simulink model "SoC_Estimation_UKF_2RC"  (R2022b)
settings: Solver=FixedStepAuto  StartTime=0.0  StopTime=time(end)  FixedStep=0.1  MaxStep=1e-2  MinStep=1e-3  RelTol=1e-3
InitFcn:
  | %% Load Dataset
  | if(exist("Battery","var")==0 && exist("SOC_LUT","var")==0)
  | clc; clear variables;
  | [file,folder]=uigetfile('*.*','Select Data File');
  | path=fullfile(folder,file);
  | load(path);
  | if(exist("Robot","var")==1)
  |     Battery=Robot;
  | elseif(exist("meas","var")==1)
  |     Battery=meas;
  |     Battery.Capacity = 2.9;
  | end
  | 
  | 
  | [time, Ia, Ic] = unique(Battery.Time); % Delete duplicate time
  | voltage = Battery.Voltage(Ia);
  | current = Battery.Current(Ia);
  | Ah = Battery.Ah(Ia);
  | if(Ah(end)<0)
  |     Ah=-Ah;
  | end
  | if(mean(current)<0)
  | current = -current; % Discharge current must be positive
  | end
  | SOC_REAL = 1-Ah/Battery.Capacity; % Discharge current must be positive
  | 
  | initialPoint=1;
  | %% Load Parameters
  | [file,folder]=uigetfile('*.*','Select Parameter File');
  | path=fullfile(folder,file);
  | load(path);
  | end
model workspace (MAT data in the model file):
  R = 1.00050162835
values from neighbouring files (symbols this model uses):
  C1 = [118829.925056 7679.67487496 914.032998183 995.696239615 1030.86324658 8477.81093389 1000000 8701.64070127 913.695760467 229.654526583]    [LFP_2RC_Parameters_PSO_13_10_2023_17_30.mat]    (also in LFP_2RC_Parameters_PSO_18_10_2023_15_27.mat = [374.526915394 91616.0371283 413980.590037 980.096839909 464; LFP_2RC_Parameters_PSO_18_10_2023_15_38.mat = [146.566073865 937.05567026 992.511993063 1291.92677117 1452; LFP_2RC_Parameters_PSO_18_10_2023_15_46.mat = [4572764.90937 926.813715587 992.544001108 773.772276009 111; NMC_2RC_Parameters_PSO_11_09_2023_10_18.mat = [27.3638316243 1000 21.9335529229 1000 31.8018075879 26.2311)
  C2 = [7193.14418842 3500000 13830.314823 10815.547426 12725.8630835 2986560.60044 129.09603881 93182.2545509 10234.9855741 3500000]    [LFP_2RC_Parameters_PSO_13_10_2023_17_30.mat]    (also in LFP_2RC_Parameters_PSO_18_10_2023_15_27.mat = [8152.77757794 7772.75056844 32340.9237315 10784.3399167 103; LFP_2RC_Parameters_PSO_18_10_2023_15_38.mat = [5380.51009562 16240.5476942 16189.4861318 10368.8792756 134; LFP_2RC_Parameters_PSO_18_10_2023_15_46.mat = [5339.98210013 16310.3382976 16188.61063 8488.61060912 12765; NMC_2RC_Parameters_PSO_11_09_2023_10_18.mat = [1323.01639542 100 1413.11035886 100 1348.21886578 1246.8775)
  OCV = [12.860136 13.025615 13.131995 13.155635 13.161545 13.173365 13.232465 13.309296 13.309296 13.604795]    [LFP_2RC_Parameters_PSO_13_10_2023_17_30.mat]    (also in LFP_2RC_Parameters_PSO_18_10_2023_15_27.mat; LFP_2RC_Parameters_PSO_18_10_2023_15_38.mat; LFP_2RC_Parameters_PSO_18_10_2023_15_46.mat; NMC_2RC_Parameters_PSO_11_09_2023_10_18.mat = [3.21503 3.23112 3.23691 3.33792 3.34178 3.34436 3.345 3.366)
  R1 = [0.001 0.113528547574 0.0897221455408 0.0815153824808 0.073763090009 0.0722149483866 0.001 0.114920856231 0.0843574753205 0.170448149157]    [LFP_2RC_Parameters_PSO_13_10_2023_17_30.mat]    (also in LFP_2RC_Parameters_PSO_18_10_2023_15_27.mat = [0.130840731393 0.001 0.001 0.0812887278858 0.0893662319552 ; LFP_2RC_Parameters_PSO_18_10_2023_15_38.mat = [0.125407853943 0.106716849555 0.100754450021 0.077403767946; LFP_2RC_Parameters_PSO_18_10_2023_15_46.mat = [1e-05 0.107896547406 0.100751200842 0.0796558546904 0.06941; NMC_2RC_Parameters_PSO_11_09_2023_10_18.mat = [0.0786652045966 0.0830695574623 0.102018078057 0.0293575040)
  R2 = [0.327796783258 0.001 0.0807740022148 0.121640548886 0.0769058248858 0.001 0.248251890874 0.001 0.101537896805 0.001]    [LFP_2RC_Parameters_PSO_13_10_2023_17_30.mat]    (also in LFP_2RC_Parameters_PSO_18_10_2023_15_27.mat = [0.32439345834 0.113786678529 0.108222017066 0.121707134426 ; LFP_2RC_Parameters_PSO_18_10_2023_15_38.mat = [0.650495945143 0.197605258421 0.107392740699 0.095938803423; LFP_2RC_Parameters_PSO_18_10_2023_15_46.mat = [0.655432908645 0.19766392139 0.107391796285 0.103804820932 ; NMC_2RC_Parameters_PSO_11_09_2023_10_18.mat = [0.155221398827 0.0699206176425 0.18163313418 0.019432263083)
  Rt = [0.226652153247 0.225527584096 0.15909738837 0.148852656484 0.143946466873 0.188428407135 0.001 0.211746487785 0.13044097603 0.184475294934]    [LFP_2RC_Parameters_PSO_13_10_2023_17_30.mat]    (also in LFP_2RC_Parameters_PSO_18_10_2023_15_27.mat = [0.109760248591 0.225130502849 0.260964397417 0.148857487521; LFP_2RC_Parameters_PSO_18_10_2023_15_38.mat = [0.0991776836505 0.174037973313 0.155548900057 0.15434594036; LFP_2RC_Parameters_PSO_18_10_2023_15_46.mat = [0.222188102228 0.173070428684 0.155550513123 0.142559241614; NMC_2RC_Parameters_PSO_11_09_2023_10_18.mat = [0.0538374601523 0.0958739914905 0.0468761371301 0.053958081)
  SOC_INTP = 0:1/66:1    [Pestimation_PSO.m]
  SOC_LUT = [0.242928992505 0.325332427039 0.408229233889 0.491515232404 0.575389970179 0.659581229809 0.744212711848 0.829280881109 0.914612975737 1]    [LFP_2RC_Parameters_PSO_13_10_2023_17_30.mat]    (also in LFP_2RC_Parameters_PSO_18_10_2023_15_27.mat; LFP_2RC_Parameters_PSO_18_10_2023_15_38.mat; LFP_2RC_Parameters_PSO_18_10_2023_15_46.mat; NMC_2RC_Parameters_PSO_11_09_2023_10_18.mat = [0.0458068965517 0.0486103448276 0.0499965517241 0.090272413)
libraries: sharedTrackingLibrary x1
settings Model: Creator=monsalve  LastModifiedBy=monsalve
settings DataIOCC: ExternalInput=[time, current],[time,voltage], [time, Ah]  LoadExternalInput=on
settings DebuggingCC: UnconnectedInputMsg=warning  UnconnectedOutputMsg=warning  UnconnectedLineMsg=warning
settings ModelReferenceCC: EnableRefExpFcnMdlSchedulingChecks=on
settings RTWCC: DLArmComputeVersion=19.05

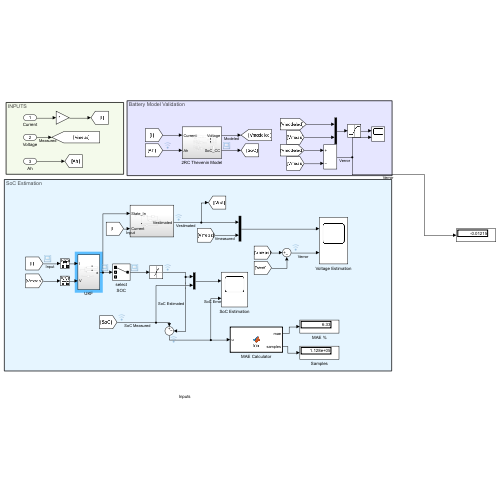
[thumbnail: Simulink's stored preview of the top-level diagram]
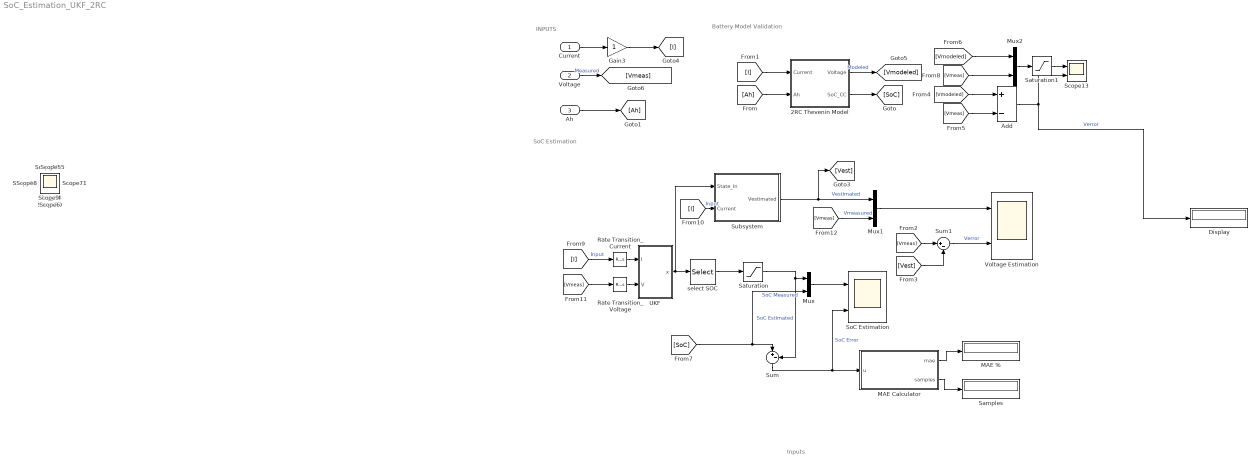
== system SoC_Estimation_UKF_2RC ==
  note: Inputs
  note: INPUTS
  note: Battery Model Validation
  note: SoC Estimation
  Current : Inport
  Voltage : Inport  Port=2
  Ah : Inport  Port=3
  2RC Thevenin Model : Subsystem
  Add : Sum  Inputs=+-
  Display : Display
  Gain3 : Gain
  MAE % : Display
  MAE Calculator : MATLAB Function  TreatAsAtomicUnit=on
  Mux : Mux  Inputs=2
  Mux1 : Mux  Inputs=2
  Mux2 : Mux  Inputs=2
  Rate Transition_Current : RateTransition  OutPortSampleTime=0.1
  Rate Transition_Voltage : RateTransition  InitialCondition=12  OutPortSampleTime=0.1
  Samples : Display
  Saturation : Saturate  UpperLimit=1  LowerLimit=0
  Saturation1 : Saturate  UpperLimit=5
  Scope13 : Scope  NumInputPorts=2
  SoC Estimation : Scope  NumInputPorts=2
  Subsystem : Subsystem
  Sum : Sum  Inputs=|+-
  Sum1 : Sum  Inputs=|+-
  UKF : Subsystem
  Voltage Estimation : Scope  NumInputPorts=2
  select SOC : Selector  InputPortWidth=3  IndexOptions=Index vector (dialog)  Indices=1  OutputSizes=1
  Scope{,1..12,14..21} (21 alike) : Scope
  wires:
  Rate Transition_Voltage/1 -> UKF/2(V)
  UKF/1(x) -> select SOC/1, Subsystem/1(State_In)
  select SOC/1 -> Saturation/1
  Sum/1 -> SoC Estimation/2, MAE Calculator/1(u)  "SoC Error"
  Mux1/1 -> Voltage Estimation/1
  Mux/1 -> SoC Estimation/1
  Saturation/1 -> Mux/1, Sum/2  "SoC Estimated"
  [I] -> Subsystem/2(Current)  "Input"
  MAE Calculator/1(mae) -> MAE %/1
  MAE Calculator/2(samples) -> Samples/1
  Subsystem/1(Vestimated) -> Mux1/1, [Vest]  "Vestimated"
  [Vmeas] -> Mux1/2  "Vmeasured"
  [Vmeas] -> Sum1/1
  [Vest] -> Sum1/2
  Sum1/1 -> Voltage Estimation/2  "Verror"
  [SoC] -> Sum/1, Mux/2  "SoC Measured"
  Rate Transition_Current/1 -> UKF/1(I)
  [Vmeas] -> Rate Transition_Voltage/1
  2RC Thevenin Model/1(Voltage) -> [Vmodeled]  "Modeled"
  [I] -> 2RC Thevenin Model/1(Current)
  Current/1 -> Gain3/1
  Gain3/1 -> [I]
  [Vmodeled] -> Add/1
  Mux2/1 -> Saturation1/1
  Voltage/1 -> [Vmeas]  "Measured"
  [Vmeas] -> Add/2
  [Vmodeled] -> Mux2/1
  2RC Thevenin Model/2(SoC_CC) -> [SoC]
  [Vmeas] -> Mux2/2
  Ah/1 -> [Ah]
  [Ah] -> 2RC Thevenin Model/2(Ah)
  [I] -> Rate Transition_Current/1  "Input"
  Add/1 -> Scope13/2, Display/1  "Verror"
  Saturation1/1 -> Scope13/1

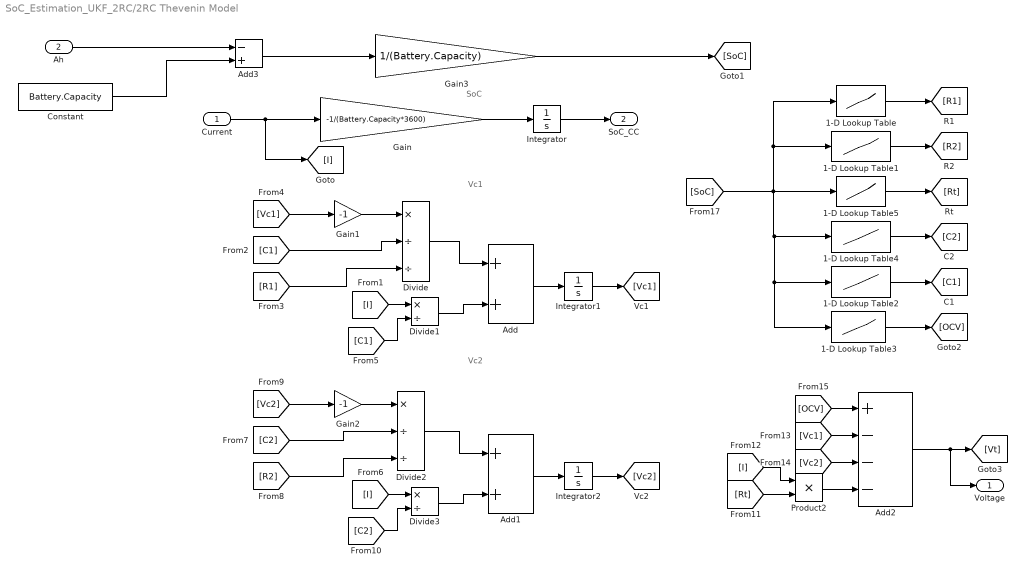
== system SoC_Estimation_UKF_2RC/2RC Thevenin Model ==
  note: Vc1
  note: SoC
  note: Vc2
  Current : Inport
  Ah : Inport  Port=2
  1-D Lookup Table : Lookup_n-D  NumberOfTableDimensions=1  BreakpointsForDimension1=SOC_LUT  Table=R1  InternalRulePriority=Speed  RndMeth=Simplest
  1-D Lookup Table1 : Lookup_n-D  NumberOfTableDimensions=1  BreakpointsForDimension1=SOC_LUT  Table=R2  InternalRulePriority=Speed  RndMeth=Simplest
  1-D Lookup Table2 : Lookup_n-D  NumberOfTableDimensions=1  BreakpointsForDimension1=SOC_LUT  Table=C1  InternalRulePriority=Speed  RndMeth=Simplest
  1-D Lookup Table3 : Lookup_n-D  NumberOfTableDimensions=1  BreakpointsForDimension1=SOC_INTP  Table=OCV  InternalRulePriority=Speed  RndMeth=Simplest
  1-D Lookup Table4 : Lookup_n-D  NumberOfTableDimensions=1  BreakpointsForDimension1=SOC_LUT  Table=C2  InternalRulePriority=Speed  RndMeth=Simplest
  1-D Lookup Table5 : Lookup_n-D  NumberOfTableDimensions=1  BreakpointsForDimension1=SOC_LUT  Table=Rt  InternalRulePriority=Speed  RndMeth=Simplest
  Add : Sum
  Add1 : Sum
  Add2 : Sum  Inputs=+---
  Add3 : Sum  Inputs=-+
  Constant : Constant  Value=Battery.Capacity
  Divide : Product  Inputs=*//
  Divide1 : Product  Inputs=*/
  Divide2 : Product  Inputs=*//
  Divide3 : Product  Inputs=*/
  Gain : Gain  Gain=-1/(Battery.Capacity*3600)
  Gain1 : Gain  Gain=-1
  Gain2 : Gain  Gain=-1
  Gain3 : Gain  Gain=1/(Battery.Capacity)
  Integrator : Integrator  InitialCondition=1  LimitOutput=on  UpperSaturationLimit=1  LowerSaturationLimit=0
  Integrator1 : Integrator
  Integrator2 : Integrator
  Product2 : Product
  Voltage : Outport
  SoC_CC : Outport  Port=2
  wires:
  Product2/1 -> Add2/4
  Add1/1 -> Integrator2/1
  1-D Lookup Table4/1 -> [C2]
  [SoC] -> 1-D Lookup Table3/1, 1-D Lookup Table2/1, 1-D Lookup Table4/1, 1-D Lookup Table5/1, 1-D Lookup Table1/1, 1-D Lookup Table/1
  [OCV] -> Add2/1
  [R1] -> Divide/3
  Divide1/1 -> Add/2
  Integrator2/1 -> [Vc2]
  [Vc1] -> Gain1/1
  Divide3/1 -> Add1/2
  Add/1 -> Integrator1/1
  Divide/1 -> Add/1
  1-D Lookup Table/1 -> [R1]
  Gain/1 -> Integrator/1
  [I] -> Divide3/1
  1-D Lookup Table3/1 -> [OCV]
  1-D Lookup Table2/1 -> [C1]
  [Vc2] -> Add2/3
  [C2] -> Divide2/2
  [Rt] -> Product2/2
  Add2/1 -> Voltage/1, [Vt]
  [I] -> Divide1/1
  [I] -> Product2/1
  Divide2/1 -> Add1/1
  [R2] -> Divide2/3
  1-D Lookup Table5/1 -> [Rt]
  Current/1 -> [I], Gain/1
  [C1] -> Divide/2
  [C2] -> Divide3/2
  1-D Lookup Table1/1 -> [R2]
  Gain2/1 -> Divide2/1
  [Vc2] -> Gain2/1
  Gain1/1 -> Divide/1
  [Vc1] -> Add2/2
  Integrator1/1 -> [Vc1]
  Integrator/1 -> SoC_CC/1
  [C1] -> Divide1/2
  Ah/1 -> Add3/1
  Add3/1 -> Gain3/1
  Constant/1 -> Add3/2
  Gain3/1 -> [SoC]

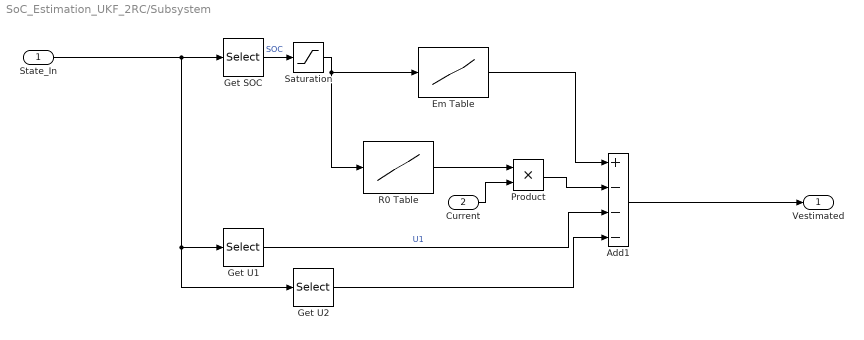
== system SoC_Estimation_UKF_2RC/Subsystem ==
  State_In : Inport
  Current : Inport  Port=2
  Add1 : Sum  Inputs=+---
  Em Table : Lookup_n-D  NumberOfTableDimensions=1  BreakpointsForDimension1=SOC_LUT  BreakpointsForDimension2=Battery.Temperature_LUT  Table=OCV  InternalRulePriority=Speed  RndMeth=Simplest
  Get SOC : Selector  InputPortWidth=3  IndexOptions=Index vector (dialog)  Indices=[1]  OutputSizes=1
  Get U1 : Selector  InputPortWidth=3  IndexOptions=Index vector (dialog)  Indices=2  OutputSizes=1
  Get U2 : Selector  InputPortWidth=3  IndexOptions=Index vector (dialog)  Indices=3  OutputSizes=1
  Product : Product
  R0 Table : Lookup_n-D  NumberOfTableDimensions=1  BreakpointsForDimension1=SOC_LUT  BreakpointsForDimension2=Battery.Temperature_LUT  Table=Rt  InternalRulePriority=Speed  RndMeth=Simplest
  Saturation : Saturate  UpperLimit=1  LowerLimit=0
  Vestimated : Outport
  wires:
  Current/1 -> Product/2
  R0 Table/1 -> Product/1
  Get U2/1 -> Add1/4
  Product/1 -> Add1/2
  Get U1/1 -> Add1/3  "U1"
  Em Table/1 -> Add1/1
  State_In/1 -> Get U2/1, Get U1/1, Get SOC/1
  Get SOC/1 -> Saturation/1  "SOC"
  Add1/1 -> Vestimated/1
  Saturation/1 -> R0 Table/1, Em Table/1

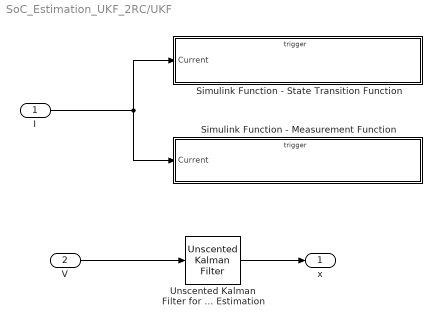
== system SoC_Estimation_UKF_2RC/UKF ==
  I : Inport
  V : Inport  Port=2
  Simulink Function - Measurement Function : Subsystem  TreatAsAtomicUnit=on
  Simulink Function - State Transition Function : Subsystem  TreatAsAtomicUnit=on
  Unscented Kalman Filter for SOC Estimation : sharedTrackingLibrary/Unscented Kalman Filter  StateTransitionFcn=batteryStateFcn  HasAdditiveProcessNoise=Additive  ProcessNoise=diag([1e-8,1e-8,1e-8])  HasTimeVaryingProcessNoise=off  HasStateTransitionFcnExtraArgument=0  InitialState=[1, 0, 0]  InitialStateCovariance=diag([1e-5,1,1])  Alpha=1  Beta=2  Kappa=0  MeasurementFcn1=batteryMeasurementFcn  HasMeasurementEnablePort1=off  HasAdditiveMeasurementNoise1=Additive  MeasurementNoise1=1  HasTimeVaryingMeasurementNoise1=off  HasMeasurementFcnExtraArgument1=0  HasMeasurementWrapping1=off  MeasurementFcn2=myMeasurementFcn  HasMeasurementEnablePort2=off  HasAdditiveMeasurementNoise2=Additive  MeasurementNoise2=1  HasTimeVaryingMeasurementNoise2=off  HasMeasurementFcnExtraArgument2=0  HasMeasurementWrapping2=off  MeasurementFcn3=myMeasurementFcn  HasMeasurementEnablePort3=off  HasAdditiveMeasurementNoise3=Additive  MeasurementNoise3=1  HasTimeVaryingMeasurementNoise3=off  HasMeasurementFcnExtraArgument3=0  HasMeasurementWrapping3=off  MeasurementFcn4=myMeasurementFcn  HasMeasurementEnablePort4=off  HasAdditiveMeasurementNoise4=Additive  MeasurementNoise4=1  HasTimeVaryingMeasurementNoise4=off  HasMeasurementFcnExtraArgument4=0  HasMeasurementWrapping4=off  MeasurementFcn5=myMeasurementFcn  HasMeasurementEnablePort5=off  HasAdditiveMeasurementNoise5=Additive  MeasurementNoise5=1  HasTimeVaryingMeasurementNoise5=off  HasMeasurementFcnExtraArgument5=0  HasMeasurementWrapping5=off  EnableMultirate=off  StateTransitionFcnSampleTime=-1  MeasurementFcn1SampleTime=-1  MeasurementFcn2SampleTime=-1  MeasurementFcn3SampleTime=-1  MeasurementFcn4SampleTime=-1  MeasurementFcn5SampleTime=-1  UseCurrentEstimator=on  OutputStateCovariance=off  DataType=double  SampleTime=0.1  NumberOfMeasurements=1
  x : Outport  VectorParamsAs1DForOutWhenUnconnected=off
  wires:
  I/1 -> Simulink Function - Measurement Function/1(Current), Simulink Function - State Transition Function/1(Current)
  V/1 -> Unscented Kalman Filter for SOC Estimation/1
  Unscented Kalman Filter for SOC Estimation/1 -> x/1

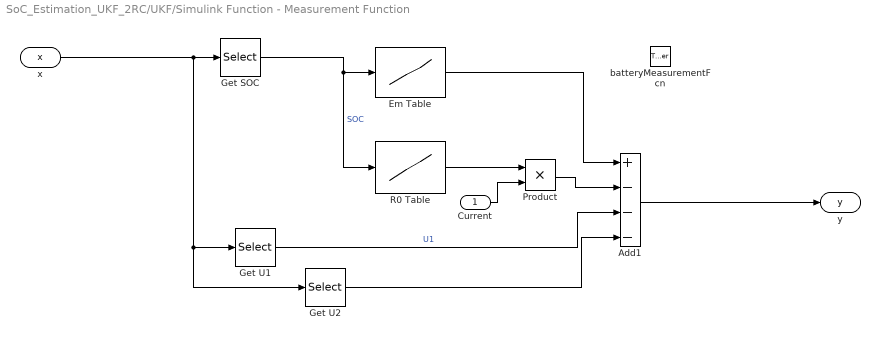
== system SoC_Estimation_UKF_2RC/UKF/Simulink Function - Measurement Function ==
  Current : Inport
  batteryMeasurementFcn : TriggerPort  TriggerType=function-call  IsSimulinkFunction=on  FunctionName=batteryMeasurementFcn  VariantControl=Variant
  Add1 : Sum  Inputs=+---
  Em Table : Lookup_n-D  NumberOfTableDimensions=1  BreakpointsForDimension1=SOC_LUT  BreakpointsForDimension2=Battery.Temperature_LUT  Table=OCV  InternalRulePriority=Speed  RndMeth=Simplest
  Get SOC : Selector  InputPortWidth=3  IndexOptions=Index vector (dialog)  Indices=[1]  OutputSizes=1
  Get U1 : Selector  InputPortWidth=3  IndexOptions=Index vector (dialog)  Indices=2  OutputSizes=1
  Get U2 : Selector  InputPortWidth=3  IndexOptions=Index vector (dialog)  Indices=3  OutputSizes=1
  Product : Product
  R0 Table : Lookup_n-D  NumberOfTableDimensions=1  BreakpointsForDimension1=SOC_LUT  BreakpointsForDimension2=Battery.Temperature_LUT  Table=Rt  InternalRulePriority=Speed  RndMeth=Simplest
  x : ArgIn  DisableCoverage=on  PortDimensions=3  ArgumentName=x
  y : ArgOut  DisableCoverage=on  ArgumentName=y
  wires:
  x/1 -> Get U2/1, Get U1/1, Get SOC/1
  Get SOC/1 -> R0 Table/1, Em Table/1  "SOC"
  Em Table/1 -> Add1/1
  R0 Table/1 -> Product/1
  Current/1 -> Product/2
  Product/1 -> Add1/2
  Get U1/1 -> Add1/3  "U1"
  Get U2/1 -> Add1/4
  Add1/1 -> y/1

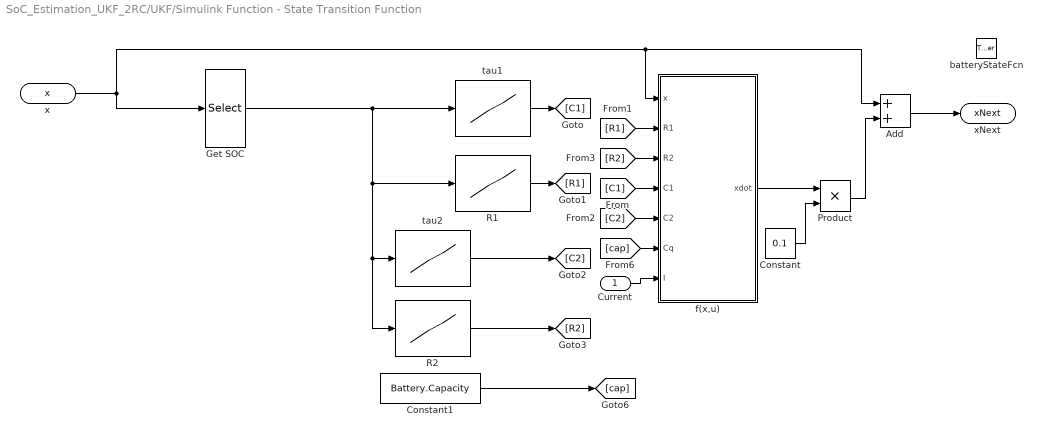
== system SoC_Estimation_UKF_2RC/UKF/Simulink Function - State Transition Function ==
  Current : Inport
  batteryStateFcn : TriggerPort  TriggerType=function-call  IsSimulinkFunction=on  FunctionName=batteryStateFcn  VariantControl=Variant
  Add : Sum
  Constant : Constant  Value=0.1
  Constant1 : Constant  Value=Battery.Capacity
  Get SOC : Selector  InputPortWidth=3  IndexOptions=Index vector (dialog)  Indices=1  OutputSizes=1
  Product : Product
  R1 : Lookup_n-D  NumberOfTableDimensions=1  BreakpointsForDimension1=SOC_LUT  BreakpointsForDimension2=Battery.Temperature_LUT  Table=R1  InternalRulePriority=Speed  RndMeth=Simplest
  R2 : Lookup_n-D  NumberOfTableDimensions=1  BreakpointsForDimension1=SOC_LUT  BreakpointsForDimension2=Battery.Temperature_LUT  Table=R2  InternalRulePriority=Speed  RndMeth=Simplest
  f(x,u) : MATLAB Function  TreatAsAtomicUnit=on
  tau1 : Lookup_n-D  NumberOfTableDimensions=1  BreakpointsForDimension1=SOC_LUT  BreakpointsForDimension2=Battery.Temperature_LUT  Table=C1  InternalRulePriority=Speed  RndMeth=Simplest
  tau2 : Lookup_n-D  NumberOfTableDimensions=1  BreakpointsForDimension1=SOC_LUT  BreakpointsForDimension2=Battery.Temperature_LUT  Table=C2  InternalRulePriority=Speed  RndMeth=Simplest
  x : ArgIn  DisableCoverage=on  PortDimensions=3  ArgumentName=x
  xNext : ArgOut  DisableCoverage=on  PortDimensions=3  ArgumentName=xNext
  wires:
  x/1 -> Get SOC/1, f(x,u)/1(x), Add/1
  Add/1 -> xNext/1
  Constant/1 -> Product/2
  f(x,u)/1(xdot) -> Product/1
  Product/1 -> Add/2
  tau1/1 -> [C1]
  [C1] -> f(x,u)/4(C1)
  R1/1 -> [R1]
  [R1] -> f(x,u)/2(R1)
  tau2/1 -> [C2]
  [C2] -> f(x,u)/5(C2)
  R2/1 -> [R2]
  [R2] -> f(x,u)/3(R2)
  Current/1 -> f(x,u)/7(I)
  Constant1/1 -> [cap]
  [cap] -> f(x,u)/6(Cq)
  Get SOC/1 -> R1/1, R2/1, tau2/1, tau1/1

== matlab function SoC_Estimation_UKF_2RC/MAE Calculator ==
  settings: updateMethod=DISCRETE
  data: u input; mae output; samples output
function [mae,samples]= fcn(u)
persistent sum i
if(isempty(sum))
    sum=abs(u);
    i=1;
else
    i=i+1;
    sum=sum+abs(u);
    
end
    
mae = sum/i*100;
samples=i;

== matlab function SoC_Estimation_UKF_2RC/UKF/Simulink Function - State Transition Function/f(x,u) ==
  data: x input; R1 input; R2 input; C1 input; C2 input; Cq input; I input; xdot output
function xdot = fx(x,R1,R2,C1,C2,Cq,I)
xdot = zeros(size(x));
U1 = x(2);
U2 = x(3);
xdot(1) = -I/(3600*Cq);
xdot(2) = -1/(C1*R1)*U1 + I/(C1);
xdot(3) = -1/(C2*R2)*U2 + I/(C2);
